simulink model "my_system"  (R2021b)
settings: Solver=FixedStepDiscrete  StartTime=0.0  StopTime=100  FixedStep=0.001  RelTol=1e-3
settings Model: Creator=lywan  LastModifiedBy=lywan
settings DataIOCC: ExternalInput=[v, x]
settings OptimizationCC: ZeroExternalMemoryAtStartup=off  ZeroInternalMemoryAtStartup=off
settings RTWCC: GenCodeOnly=on  TargetLang=C++
settings GRTTargetCC: TargetLangStandard=C++11 (ISO)  CodeInterfacePackaging=C++ class

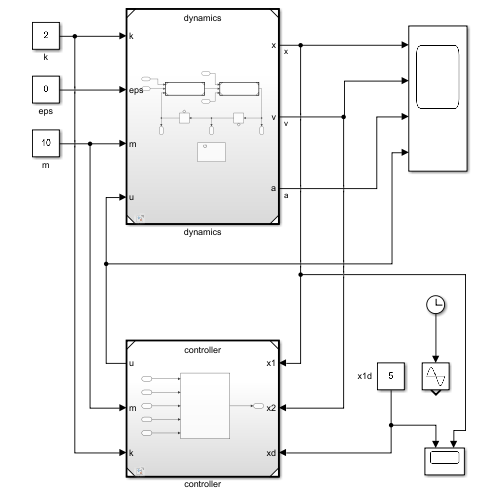
[thumbnail: Simulink's stored preview of the top-level diagram]
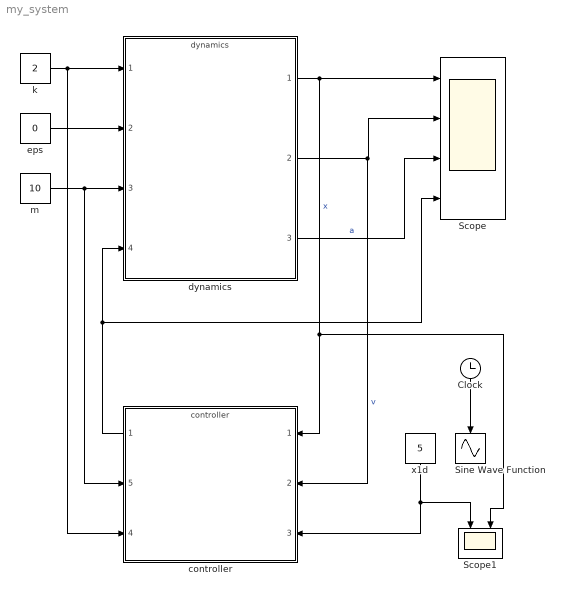
== system my_system ==
  Clock : Clock
  Scope : Scope  NumInputPorts=4
  Scope1 : Scope  NumInputPorts=2
  Sine Wave Function : Sin  TimeSource=Use external signal  Amplitude=3  Frequency=0.2  SampleTime=0
  controller : ModelReference  ModelNameDialog=controller.slx  SimulationMode=Normal  ModelReferenceVersion=1.6
      settings: PortSchema="{\"entries\":[{\"content\":{\"sides\":[{\"content\":{\"connectorIds\":[\"In1\",\"In2\",\"In3\"]},\"type\":\"ConnectorPlacement.EquallySpacedRectSide\",\"uuid\":\"6012a128-6580-457e-a822-c0faca2527c1\"},{\"content\":{\"connectorIds\":[\"Out1\",\"In5\",\"In4\"],\"side\":\"RIGHT\"},\"type\":\"ConnectorPlacement.EquallySpacedRectSide\",\"uuid\":\"22ade6ac-eebd-4cf5-8199-4f654f112887\"},{\"content\":{\"connectorIds\":[],\"side\":\"TOP\"},\"type\":\"ConnectorPlacement.EquallySpacedRectSide\",\"uuid\":\"453940ff-35dc-4844-8393-5e9d30328de3\"}]},\"type\":\"ConnectorPlacement.EquallySpacedConnector\",\"uuid\":\"db50fdd7-a1e1-4e7d-bbb2-33e79fdbae12\"}],\"packageUris\":[\"http://schema.mathworks.com/mf0/Connector/R2020b\"],\"version\":\"1.0\"}"
  dynamics : ModelReference  ModelNameDialog=dynamics.slx  SimulationMode=Normal  ModelReferenceVersion=1.54
  eps : Constant  Value=0
  k : Constant  Value=2
  m : Constant  Value=10
  x1d : Constant  Value=5
  wires:
  eps/1 -> dynamics/2
  k/1 -> dynamics/1, controller/4
  m/1 -> dynamics/3, controller/5
  Clock/1 -> Sine Wave Function/1
  dynamics/1 -> Scope1/2, controller/1, Scope/1  "x"
  dynamics/2 -> controller/2, Scope/2  "v"
  dynamics/3 -> Scope/3  "a"
  controller/1 -> Scope/4, dynamics/4
  x1d/1 -> Scope1/1, controller/3
